simulink library "starslibGeodesy"  (R2022b)
settings: Solver=ode45  StartTime=0.0  StopTime=10.0  RelTol=1e-3  EnableMultiTasking=on
undefined symbols (not defined in the file): SimIn
libraries: $bdroot x6, starslibMathOperations x3, simulink x1, starslibAxisTransformations x1
settings Model: Creator=eheim  LastModifiedBy=macheson
settings SolverCC: AlgebraicLoopSolver=TrustRegion
settings DataIOCC: LimitDataPoints=on  SaveFormat=Array  SignalLoggingSaveFormat=ModelDataLogs  ReturnWorkspaceOutputs=off
settings OptimizationCC: ExpressionDepthLimit=2147483647  LifeSpan=inf
settings DebuggingCC: UnderspecifiedInitializationDetection=Classic  MergeDetectMultiDrivingBlocksExec=none  SolverPrmCheckMsg=warning  FcnCallInpInsideContextMsg=warning  UnconnectedInputMsg=warning  UnconnectedOutputMsg=warning  UnconnectedLineMsg=warning  StateNameClashWarn=warning  SFUnexpectedBacktrackingDiag=warning  SFNoUnconditionalDefaultTransitionDiag=warning  SFExecutionAtInitializationDiag=none  SFMachineParentedDataDiag=warning  ArithmeticOperatorsInVariantConditions=warning
settings HardwareCC: ProdBitPerPointer=32  ProdBitPerSizeT=32  ProdBitPerPtrDiffT=32  ProdLargestAtomicFloat=None  ProdIntDivRoundTo=Undefined  ProdEndianess=Unspecified  ProdWordSize=32  ProdHWDeviceType=32-bit Generic
settings ModelReferenceCC: PropagateSignalLabelsOutOfModel=off
settings SFSimCC: SimUseLocalCustomCode=off  CustomCodeUndefinedFunction=UseInterfaceOnly
settings RTWCC: RTWUseLocalCustomCode=off
settings CodeAppCC: StateflowObjectComments=on
settings GRTTargetCC: TargetLangStandard=C89/C90 (ANSI)  CombineOutputUpdateFcns=off  GRTInterface=on
settings ConfigComp: CovMetricSettings=dw  CovSaveCumulativeToWorkspaceVar=on  CovSaveSingleToWorkspaceVar=on  CovExternalEMLEnable=off  CovSFcnEnable=off

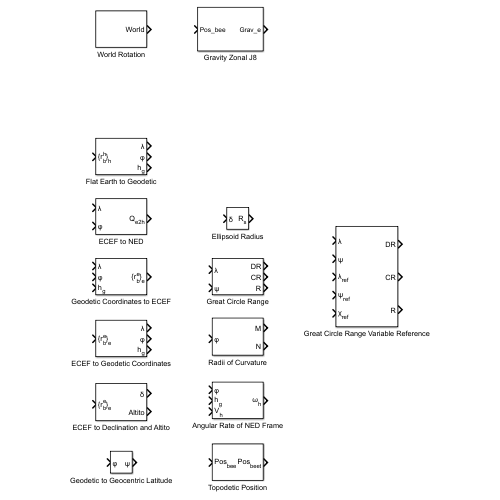
[thumbnail: Simulink's stored preview of the top-level diagram]
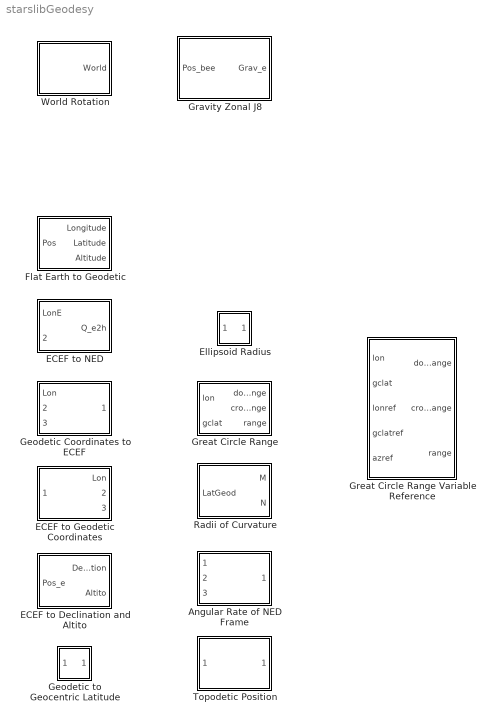
== system starslibGeodesy ==
  Angular Rate of NED Frame : Subsystem  mask(Angular Rate of NED Frame){a=SimIn.Environment.Earth.RadiusEquator, e=SimIn.Environment.Earth.Eccentricity}
      mask prompts: a "Semi-major axis radius"; e "Eccentricity"
      mask help: Computes the angular rate of the local North-East-Down frame.
      mask Display:
      | port_label('input',1,'\phi','texmode','on')
      | port_label('input',2,'h_g','texmode','on')
      | port_label('input',3,'V_h','texmode','on')
      | port_label('output',1,'\omega_{h}','texmode','on')
  ECEF to Declination and Altito : Subsystem  mask(Declination and Altito){a=SimIn.Environment.Earth.RadiusEquator, b=SimIn.Environment.Earth.RadiusPoles}
      mask prompts: a "Semi-major axis radius"; b "Semi-minor axis radius"
      mask help:
      | Calculates angle from equatorial plane to radius vector of vehicle from center of planet, declination and component of radius magnitude above the ellipsoid, altito.
      |
      | Note: Units of input parameters must be same as units of the ECEF position input.
      mask Display:
      | port_label('input',1,'\{r_b^e\}_e','texmode','on')
      | port_label('output',1,'\delta','texmode','on')
      | port_label('output',2,'Altito','texmode','on')
  ECEF to Geodetic Coordinates : Subsystem  mask(ECEF to LLA){a=SimIn.Environment.Earth.RadiusEquator, b=SimIn.Environment.Earth.RadiusPoles, tol=1e-12}
      mask prompts: a "Semi-major axis radius"; b "Semi-minor axis radius"; tol "Minum distance from semi-minor axis"
      mask help:
      | Calculates Longitude, Geodetic Latitude and Geodetic Altitude from Earth Centered Earth Fixed (ECEF) position.
      |
      | Note: Units of input parameters must be same as units of the ECEF position input.
      |
      | Reference:
      | Explanatory Supplement to the Astronomical Almanac
      | Edited by P. Kenneth Seidelmann, 1992
      | University Science Books
      | Sausalito, California
      mask Display:
      | port_label('input',1,'\{r_b^e\}_e','texmode','on')
      | port_label('output',1,'\lambda','texmode','on')
      | port_label('output',2,'\phi','texmode','on')
      | port_label('output',3,'h_g','texmode','on')
  ECEF to NED : Subsystem  mask(ECEF to NED){}
      mask help: Creates quaternion from ECEF axes to local North-East-Down axes by transforming through longitude and geodetic latitude.
      mask Display:
      | port_label('output',1,'Q_{e2h}','texmode','on')
      | port_label('input',1,'\lambda','texmode','on')
      | port_label('input',2,'\phi','texmode','on')
  Ellipsoid Radius : Subsystem  mask(Ellipsoid radius){a=SimIn.Environment.Earth.RadiusEquator, b=SimIn.Environment.Earth.RadiusPoles}
      mask prompts: a "Semi-major axis radius"; b "Semi-minor axis radius"
      mask help: Radius of ellipsoid at geocentric latitude or declination. If geocentric latitude is used the output is the ellipsoid radius at that geocentric latitude. If declination is used the output is then radius of ellipsoid where radius to vehicle pierces the ellipsoid. Units of radius vector are determined by units of semi-major-axis parmeter.
      mask Help:
      | Ref: E. W. PURCELL, E. W. and COWAN, W. B., Relating Geodetic Latitude and Altitude to Geocentric Latitude and Radius Vector, ARS Journal, Jan. 1961, page 934, eqn 5.
      | W. B. COWAN2
      | Aeronutronic Div., Ford Motor Co.
      | Newport Beach, Calif.
      mask Display:
      | port_label('input',1,'\delta','texmode','on')
      | port_label('output',1,'R_s','texmode','on')
  Flat Earth to Geodetic : Subsystem  mask(Flat Earth to Geodetic){lat=SimIn.IC.LatGeod, lon=SimIn.IC.Lon, a=SimIn.Environment.Earth.RadiusEquator, e=SimIn.Environment.Earth.Eccentricity}
      mask prompts: lat "Initial geodetic latitude (radians)"; lon "Initial longitude (radians)"; a "Planet semi-major axis radius"; e "Planet eccentricity"
      mask help: Estimates geodetic latitude, longitude and altitude from change in North-East-Down position. Input position units must match units of planet parmeters.
      mask Display:
      | port_label('input',1,'\{r_b^h\}_h','texmode','on')
      | port_label('output',1,'\lambda','texmode','on')
      | port_label('output',2,'\phi','texmode','on')
      | port_label('output',3,'h_g','texmode','on')
  Geodetic Coordinates to ECEF : Subsystem  mask(LLA to ECEF){a=SimIn.Environment.Earth.RadiusEquator, e=SimIn.Environment.Earth.Eccentricity}
      mask prompts: a "Semi-major axis radius"; e "Eccentricity"
      mask help: Converts geodetic latitude, longitude, and altitude to Cartesian ECEF coordinates.
      mask Display:
      | port_label('output',1,'\{r_b^e\}_e','texmode','on')
      | port_label('input',1,'\lambda','texmode','on')
      | port_label('input',2,'\phi','texmode','on')
      | port_label('input',3,'h_g','texmode','on')
  Geodetic to Geocentric Latitude : Subsystem  mask(Geodetic to Geocentric Latitude){e=SimIn.Environment.Earth.Eccentricity}
      mask prompts: e "Eccentricity"
      mask help: Converts geodetic latitude to geocentric latitude.
      mask Display:
      | port_label('input',1,'\phi','texmode','on')
      | port_label('output',1,'\psi','texmode','on')
  Gravity Zonal J8 : Subsystem  mask(Gravity Zonal J8){a=SimIn.Environment.Earth.RadiusEquator, mu=SimIn.Environment.Earth.Gravity.mu, J=SimIn.Environment.Earth.Gravity.Jcoefs}
      mask prompts: a "Semi-major axis radius"; mu "Gravitational Constant"; J "Zonal Coefficients"
      mask help: Gravity model with up to 8 zonal coefficients.
  Great Circle Range : Subsystem  mask(Great Circle Range){signconv=Positive approaching reference, lonref=SimIn.Environment.Runway.Lon, latref=SimIn.Environment.Runway.LatGeoc, Rref=SimIn.Environment.Runway.Rref, azref=SimIn.Environment.Runway.Heading, a=SimIn.Environment.Earth.RadiusEquator, b=SimIn.Environment.Earth.RadiusPoles}
      mask prompts: signconv "Downrange sign convention"; lonref "Reference Longitude (rad)"; latref "Reference Geocentric Latitude (rad)"; Rref "Refernce Ellipsoid Radius"; azref "Reference Azimuth (rad)"; a "Semi-major-axis radius"; b "Semi-minor-axis radius"
      mask help:
      | Computes downrange and cross range based on relative great circles between the reference location and the vehicle location given longitude and geocentric latitude of each and a reference azimuth.
      |
      | The refernce azimuth can be any arbitrary fixed azimuth.  For example, launch vehicles typically use the launch azimuth with downrange positive departing the reference.  Approach and landing vehicle may use the runway azimuth.
      |
      | Crossrange is defined as the perpendicular distance from the great circle of the reference azimuth to the vehicle.  Cross range is positive in the increasing azimuth direction.
      |
      | Downrange is defined as the distance along the great circle created by the reference azimuth from the reference location to the point at which the crossrange is measured from.  Downrange sign convention can be selected to be either positive when departing or positive when approaching the reference location along the reference azimuth.
      |
      | Units used for Earth radii determine units for downrange and crossrange.
      mask init:
      | switch signconv
      |     case 1
      |         signconv = 1;
      |     case 2
      |         signconv = -1;
      | end
      mask TypeOptions signconv: Positive departing reference | Positive approaching reference
      mask Display:
      | port_label('input',1,'\lambda','texmode','on')
      | port_label('input',2,'\psi','texmode','on')
      | port_label('output',1,'DR','texmode','on')
      | port_label('output',2,'CR','texmode','on')
      | port_label('output',3,'R','texmode','on')
  Great Circle Range Variable Reference : Subsystem  mask(Great Circle Range Variable Reference){signconv=Positive approaching reference, a=SimIn.Environment.Earth.RadiusEquator, b=SimIn.Environment.Earth.RadiusPoles}
      mask prompts: signconv "Downrange sign convention"; a "Semi-major-axis radius"; b "Semi-minor-axis radius"
      mask help:
      | Computes downrange and cross range based on relative great circles between the reference location and the vehicle location given longitude and geocentric latitude of each and a reference azimuth.
      |
      | The refernce azimuth can be any arbitrary azimuth.  For example, launch vehicles typically use the launch azimuth with downrange positive departing the reference.  Approach and landing vehicle may use the runway azimuth or the vehicle ground track with downrange positive approaching the reference location.
      |
      | Crossrange is defined as the perpendicular distance from the great circle of the reference azimuth to the vehicle.  Cross range is positive in the increasing azimuth direction.
      |
      | Downrange is defined as the distance along the great circle created by the reference azimuth from the reference location to the point at which the crossrange is measured from.  Downrange sign convention can be selected to be either positive when departing or positive when approaching the reference location along the reference azimuth.
      |
      | Units used for Earth radii determine units for downrange and crossrange.
      mask init:
      | switch signconv
      |     case 1
      |         signconv = 1;
      |     case 2
      |         signconv = -1;
      | end
      mask TypeOptions signconv: Positive departing reference | Positive approaching reference
      mask Display:
      | port_label('input',1,'\lambda','texmode','on')
      | port_label('input',2,'\psi','texmode','on')
      | port_label('input',3,'\lambda_{ref}','texmode','on')
      | port_label('input',4,'\psi_{ref}','texmode','on')
      | port_label('input',5,'\chi_{ref}','texmode','on')
      | 
      | port_label('output',1,'DR','texmode','on')
      | port_label('output',2,'CR','texmode','on')
      | port_label('output',3,'R','texmode','on')
  Radii of Curvature : Subsystem  mask(Radii of Curvature){a=SimIn.Environment.Earth.RadiusEquator, e=SimIn.Environment.Earth.Eccentricity}
      mask prompts: a "Semi-major axis radius"; e "Eccentricity"
      mask help: Computes the radii of curvature for the ellipsoid
      mask Display:
      | port_label('input',1,'\phi','texmode','on')
      | port_label('output',1,'M','texmode','on')
      | port_label('output',2,'N','texmode','on')
  Topodetic Position : Subsystem  mask(Topodedic Position){Pos_bee=SimIn.EOM.Pos_bee, Q_e2h=SimIn.EOM.Q_e2h}
      mask prompts: Pos_bee "Initial Position (Pos_bee)"; Q_e2h "Initial Transformation (Q_e2h)"
      mask help: NED position relative to initial NED position in initial NED coordinates.
      mask Display:
      | port_label('input' ,1,'Pos_{bee}','texmode','on')
      | port_label('output' ,1,'Pos_{bee}_t','texmode','on')
  World Rotation : Subsystem  mask(World Rotation){omega=SimIn.Environment.Earth.Omega, ERA_IC=SimIn.Environment.Earth.ERA_IC}
      mask prompts: omega "Rotation Rate"; ERA_IC "Initial Rotation Angle"
      mask help:
      | Tracks current world rotation angle and inertial orientation as simulation progresses.
      |
      | Note: The initial rotation angle is for simulation time equal to zero.
      mask Display: port_label('output', 1, 'World');

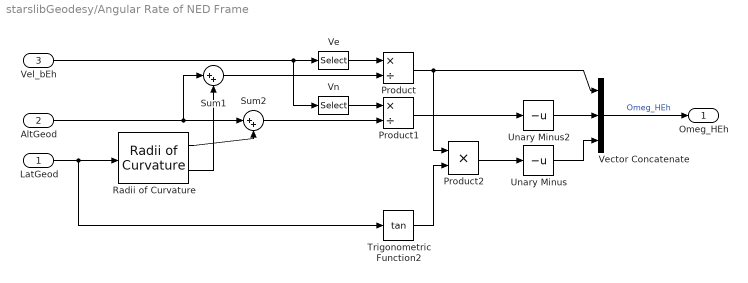
== system starslibGeodesy/Angular Rate of NED Frame ==
  LatGeod : Inport
  AltGeod : Inport  Port=2
  Vel_bEh : Inport  Port=3
  Product : Product  Inputs=*/  RndMeth=Zero
  Product1 : Product  Inputs=*/  RndMeth=Zero
  Product2 : Product  RndMeth=Zero
  Radii of Curvature : $bdroot/Radii of Curvature  a=a  e=e
  Sum1 : Sum  Inputs=|++
  Sum2 : Sum  Inputs=|++
  Trigonometric Function2 : Trigonometry  Operator=tan
  Unary Minus : UnaryMinus
  Unary Minus2 : UnaryMinus
  Ve : Selector  NumberOfDimensions=2  InputPortWidth=3  IndexOptions=Index vector (dialog),Select all  Indices=2,1  OutputSizes=1,1
  Vector Concatenate : Concatenate  NumInputs=3  Mode=Multidimensional array
  Vn : Selector  NumberOfDimensions=2  InputPortWidth=3  IndexOptions=Index vector (dialog),Select all  Indices=1,1  OutputSizes=1,1
  Omeg_HEh : Outport  PortDimensions=[3,1]
  wires:
  Vel_bEh/1 -> Vn/1, Ve/1
  LatGeod/1 -> Radii of Curvature/1, Trigonometric Function2/1
  Trigonometric Function2/1 -> Product2/2
  Vector Concatenate/1 -> Omeg_HEh/1  "Omeg_HEh"
  Product/1 -> Vector Concatenate/1, Product2/1
  Product2/1 -> Unary Minus/1
  Product1/1 -> Unary Minus2/1
  Ve/1 -> Product/1
  Vn/1 -> Product1/1
  Unary Minus2/1 -> Vector Concatenate/2
  Unary Minus/1 -> Vector Concatenate/3
  Sum1/1 -> Product/2
  Sum2/1 -> Product1/2
  Radii of Curvature/2 -> Sum1/2
  Radii of Curvature/1 -> Sum2/2
  AltGeod/1 -> Sum1/1, Sum2/1

== system starslibGeodesy/ECEF to Declination and Altito ==
  Pos_e : Inport
  Ellipsoid Radius : $bdroot/Ellipsoid Radius  a=a  b=b
  Math Function : Math  Operator=hypot  SignedPower=on
  Math Function1 : Math  Operator=hypot  SignedPower=on
  Selector : Selector  InputPortWidth=3  IndexOptions=Index vector (dialog)  Indices=3  OutputSizes=1
  Selector1 : Selector  InputPortWidth=3  IndexOptions=Index vector (dialog)  Indices=2  OutputSizes=1
  Selector2 : Selector  InputPortWidth=3  IndexOptions=Index vector (dialog)  Indices=1  OutputSizes=1
  Sum : Sum  Inputs=|+-
  Trigonometric Function3 : Trigonometry  Operator=atan2
  Declination : Outport
  Altito : Outport  Port=2
  wires:
  Sum/1 -> Altito/1  "Altito"
  Selector1/1 -> Math Function/2
  Selector2/1 -> Math Function/1
  Pos_e/1 -> Selector2/1, Selector/1, Selector1/1
  Math Function/1 -> Trigonometric Function3/2, Math Function1/2
  Selector/1 -> Trigonometric Function3/1, Math Function1/1
  Trigonometric Function3/1 -> Declination/1, Ellipsoid Radius/1  "Declination"
  Math Function1/1 -> Sum/1
  Ellipsoid Radius/1 -> Sum/2

== system starslibGeodesy/ECEF to Geodetic Coordinates ==
  note: Reference:
      | Explanatory Supplement to the Astronomical Almanac
      | Edited by P. Kenneth Seidelmann, 1992
      | University Science Books
      | Sausalito, California
  Pos_bee : Inport
  Distance to Axis : Subsystem
  Geodetic Altitude : Subsystem
  Geodetic Latitude : Subsystem
  Selector2 : Selector  InputPortWidth=3  IndexOptions=Index vector (dialog)  Indices=1  OutputSizes=1
  Selector3 : Selector  InputPortWidth=3  IndexOptions=Index vector (dialog)  Indices=2  OutputSizes=1
  Selector5 : Selector  InputPortWidth=3  IndexOptions=Index vector (dialog)  Indices=3  OutputSizes=1
  Trigonometric Function1 : Trigonometry  Operator=atan2
  t : Subsystem
  Lon : Outport
  LatGeod : Outport  Port=2
  AltGeod : Outport  Port=3
  wires:
  Trigonometric Function1/1 -> Lon/1  "Lon"
  Selector2/1 -> Trigonometric Function1/2  "X"
  Selector3/1 -> Trigonometric Function1/1  "Y"
  Geodetic Altitude/1(AltGeod) -> AltGeod/1  "AltGeod"
  Distance to Axis/1(r) -> Geodetic Altitude/2(r), t/2(r)  "r"
  Geodetic Latitude/1(LatGeod) -> LatGeod/1, Geodetic Altitude/4(LatGeod)  "LatGeod"
  Distance to Axis/2(min) -> Geodetic Latitude/3(min)
  t/1(t) -> Geodetic Altitude/3(t), Geodetic Latitude/2(t)
  Pos_bee/1 -> Selector3/1, Selector2/1, Selector5/1, Distance to Axis/1(Pos)
  Selector5/1 -> t/1(Z), Geodetic Latitude/1(Z), Geodetic Altitude/1(Z)  "Z"

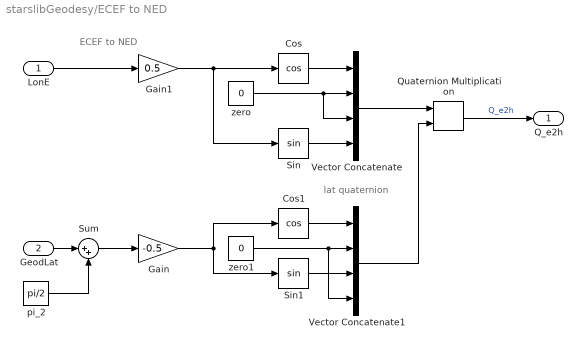
== system starslibGeodesy/ECEF to NED ==
  note: lat quaternion
  note: ECEF to NED
  LonE : Inport
  GeodLat : Inport  Port=2
  Cos : Trigonometry  Operator=cos
  Cos1 : Trigonometry  Operator=cos
  Gain : Gain  Gain=-0.5
  Gain1 : Gain  Gain=0.5
  Quaternion Multiplication : starslibMathOperations/Quaternion Multiplication  n=0
  Sin : Trigonometry
  Sin1 : Trigonometry
  Sum : Sum  Inputs=|++
  Vector Concatenate : Concatenate  NumInputs=4  Mode=Multidimensional array
  Vector Concatenate1 : Concatenate  NumInputs=4  Mode=Multidimensional array
  pi_2 : Constant  Value=pi/2
  zero : Constant  Value=0
  zero1 : Constant  Value=0
  Q_e2h : Outport
  wires:
  GeodLat/1 -> Sum/1
  LonE/1 -> Gain1/1
  Quaternion Multiplication/1 -> Q_e2h/1  "Q_e2h"
  Vector Concatenate1/1 -> Quaternion Multiplication/2
  Vector Concatenate/1 -> Quaternion Multiplication/1
  Gain/1 -> Sin1/1, Cos1/1
  Sin1/1 -> Vector Concatenate1/3
  Cos1/1 -> Vector Concatenate1/1
  Gain1/1 -> Sin/1, Cos/1
  Sin/1 -> Vector Concatenate/4
  zero/1 -> Vector Concatenate/2, Vector Concatenate/3
  Cos/1 -> Vector Concatenate/1
  Sum/1 -> Gain/1
  pi_2/1 -> Sum/2
  zero1/1 -> Vector Concatenate1/2, Vector Concatenate1/4

== system starslibGeodesy/Ellipsoid Radius ==
  Declination : Inport
  Add1 : Sum  Inputs=-+
  Add2 : Sum
  Constant1 : Constant  Value=b
  Constant2 : Constant
  Constant4 : Constant  Value=a
  Divide : Product  Inputs=*/
  Divide1 : Product  Inputs=*/
  Math Function1 : Math  Operator=square  SignedPower=on
  Math Function7 : Math  Operator=square  SignedPower=on
  Product5 : Product  RndMeth=Zero
  Sqrt : Sqrt
  Trigonometric Function : Trigonometry
  Rs : Outport
  wires:
  Trigonometric Function/1 -> Math Function7/1
  Constant2/1 -> Add1/1, Add2/1
  Add1/1 -> Product5/1
  Product5/1 -> Add2/2
  Math Function7/1 -> Product5/2
  Add2/1 -> Sqrt/1
  Sqrt/1 -> Divide/2
  Divide/1 -> Rs/1  "Rs"
  Declination/1 -> Trigonometric Function/1
  Divide1/1 -> Math Function1/1
  Math Function1/1 -> Add1/2
  Constant1/1 -> Divide1/2
  Constant4/1 -> Divide1/1, Divide/1

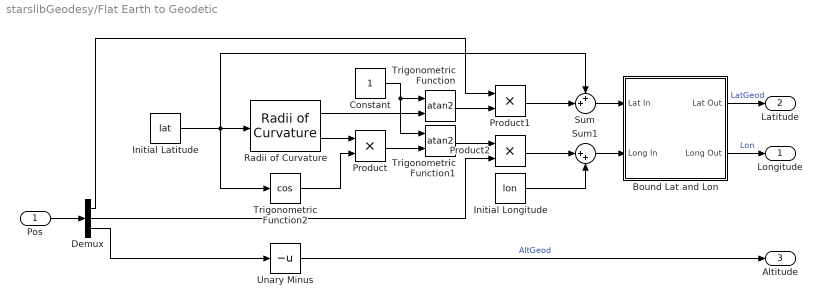
== system starslibGeodesy/Flat Earth to Geodetic ==
  Pos : Inport
  Bound Lat and Lon : Subsystem
  Constant : Constant
  Demux : Demux  Outputs=3
  Initial Latitude : Constant  Value=lat
  Initial Longitude : Constant  Value=lon
  Product : Product  RndMeth=Zero
  Product1 : Product  RndMeth=Zero
  Product2 : Product  RndMeth=Zero
  Radii of Curvature : $bdroot/Radii of Curvature  a=a  e=e
  Sum : Sum  Inputs=++|
  Sum1 : Sum  Inputs=|++
  Trigonometric Function : Trigonometry  Operator=atan2
  Trigonometric Function1 : Trigonometry  Operator=atan2
  Trigonometric Function2 : Trigonometry  Operator=cos
  Unary Minus : UnaryMinus
  Longitude : Outport
  Latitude : Outport  Port=2
  Altitude : Outport  Port=3
  wires:
  Radii of Curvature/2 -> Product/1
  Initial Latitude/1 -> Radii of Curvature/1, Trigonometric Function2/1, Sum/1
  Trigonometric Function2/1 -> Product/2
  Initial Longitude/1 -> Sum1/2
  Trigonometric Function/1 -> Product1/2
  Radii of Curvature/1 -> Trigonometric Function/2
  Constant/1 -> Trigonometric Function/1, Trigonometric Function1/1
  Product/1 -> Trigonometric Function1/2
  Trigonometric Function1/1 -> Product2/1
  Pos/1 -> Demux/1
  Demux/1 -> Product1/1
  Demux/2 -> Product2/2
  Demux/3 -> Unary Minus/1
  Unary Minus/1 -> Altitude/1  "AltGeod"
  Product1/1 -> Sum/2
  Product2/1 -> Sum1/1
  Sum/1 -> Bound Lat and Lon/1(Lat In)
  Sum1/1 -> Bound Lat and Lon/2(Long In)
  Bound Lat and Lon/1(Lat Out) -> Latitude/1  "LatGeod"
  Bound Lat and Lon/2(Long Out) -> Longitude/1  "Lon"

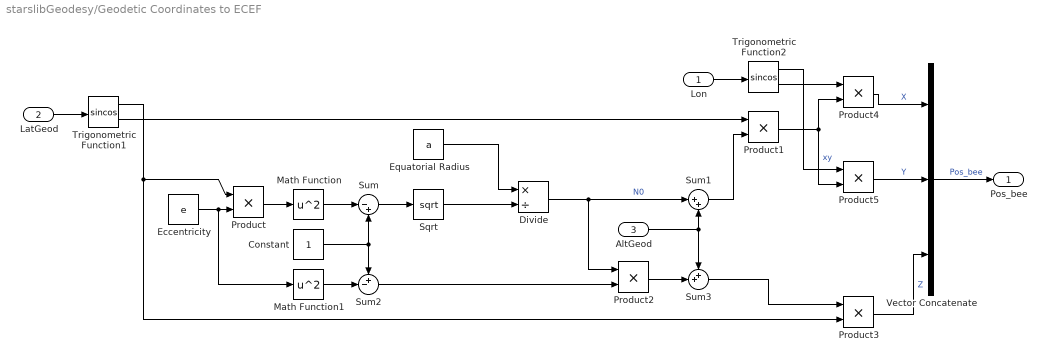
== system starslibGeodesy/Geodetic Coordinates to ECEF ==
  Lon : Inport
  LatGeod : Inport  Port=2
  AltGeod : Inport  Port=3
  Constant : Constant
  Divide : Product  Inputs=*/
  Eccentricity : Constant  Value=e
  Equatorial Radius : Constant  Value=a
  Math Function : Math  Operator=square  SignedPower=on
  Math Function1 : Math  Operator=square  SignedPower=on
  Product{,1..5} (6 alike) : Product  RndMeth=Zero
  Sqrt : Sqrt
  Sum : Sum  Inputs=|-+
  Sum1 : Sum  Inputs=|++
  Sum2 : Sum  Inputs=+-|
  Sum3 : Sum  Inputs=++|
  Trigonometric Function1 : Trigonometry  Operator=sincos
  Trigonometric Function2 : Trigonometry  Operator=sincos
  Vector Concatenate : Concatenate  NumInputs=3  Mode=Multidimensional array
  Pos_bee : Outport
  wires:
  Equatorial Radius/1 -> Divide/1
  Sqrt/1 -> Divide/2
  Eccentricity/1 -> Product/2, Math Function1/1
  Trigonometric Function1/1 -> Product/1, Product3/2
  Product/1 -> Math Function/1
  Constant/1 -> Sum/2, Sum2/1
  Math Function/1 -> Sum/1
  Sum/1 -> Sqrt/1
  Divide/1 -> Sum1/1, Product2/1  "N0"
  AltGeod/1 -> Sum1/2, Sum3/1
  Sum1/1 -> Product1/2
  Product1/1 -> Product4/2, Product5/2  "xy"
  Math Function1/1 -> Sum2/2
  Sum2/1 -> Product2/2
  LatGeod/1 -> Trigonometric Function1/1
  Trigonometric Function1/2 -> Product1/1
  Trigonometric Function2/1 -> Product5/1
  Trigonometric Function2/2 -> Product4/1
  Lon/1 -> Trigonometric Function2/1
  Product5/1 -> Vector Concatenate/2  "Y"
  Product4/1 -> Vector Concatenate/1  "X"
  Product3/1 -> Vector Concatenate/3  "Z"
  Vector Concatenate/1 -> Pos_bee/1  "Pos_bee"
  Product2/1 -> Sum3/2
  Sum3/1 -> Product3/1

== system starslibGeodesy/Geodetic to Geocentric Latitude ==
  Geodetic Latitude : Inport
  Constant : Constant
  Constant1 : Constant  Value=e
  Math Function : Math  Operator=square  SignedPower=on
  Product : Product
  Sum : Sum  Inputs=|+-
  Trigonometric Function : Trigonometry  Operator=tan
  Trigonometric Function1 : Trigonometry  Operator=atan
  Geocentric Latitude : Outport
  wires:
  Product/1 -> Trigonometric Function1/1
  Trigonometric Function/1 -> Product/1
  Trigonometric Function1/1 -> Geocentric Latitude/1
  Geodetic Latitude/1 -> Trigonometric Function/1
  Constant/1 -> Sum/1
  Sum/1 -> Product/2
  Constant1/1 -> Math Function/1
  Math Function/1 -> Sum/2

== system starslibGeodesy/Gravity Zonal J8 ==
  Pos_bee : Inport
  Constant : Constant  Value=a
  Constant1 : Constant  Value=mu
  Constant2 : Constant  Value=J
  Gravity Zonal J8 : MATLAB Function  TreatAsAtomicUnit=on
  Grav_e : Outport
  wires:
  Pos_bee/1 -> Gravity Zonal J8/1(pecef)
  Constant2/1 -> Gravity Zonal J8/4(J)
  Constant1/1 -> Gravity Zonal J8/3(mu)
  Constant/1 -> Gravity Zonal J8/2(a)
  Gravity Zonal J8/1(Grav_e) -> Grav_e/1  "Grav_e"

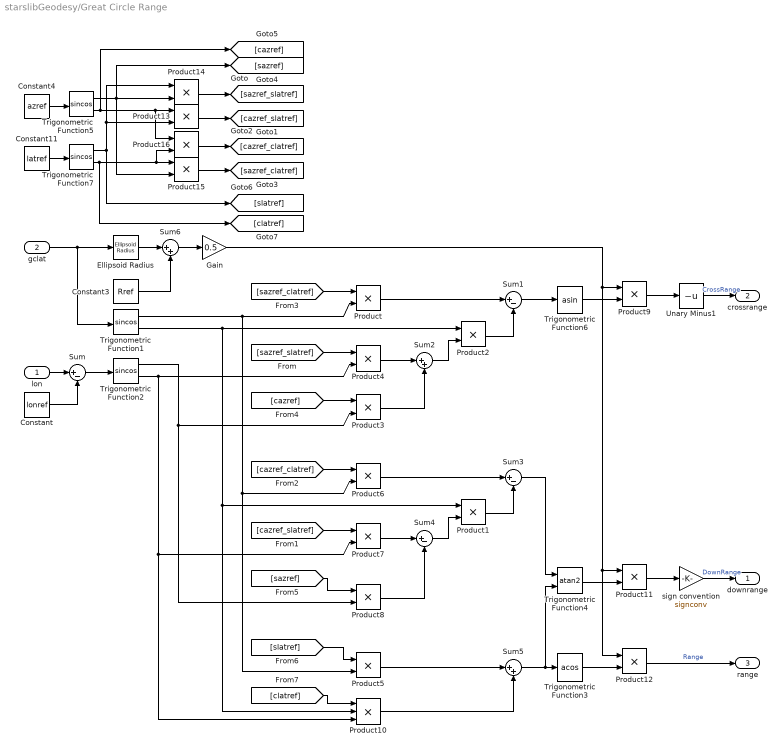
== system starslibGeodesy/Great Circle Range ==
  lon : Inport
  gclat : Inport  Port=2
  Constant : Constant  Value=lonref
  Constant11 : Constant  Value=latref
  Constant3 : Constant  Value=Rref
  Constant4 : Constant  Value=azref
  Ellipsoid Radius : $bdroot/Ellipsoid Radius  a=a  b=b
  Gain : Gain  Gain=0.5
  Product{,1..9,11..16} (16 alike) : Product  RndMeth=Zero
  Product10 : Product  Inputs=3  RndMeth=Zero
  Sum{,1,3..4} (4 alike) : Sum  Inputs=|+-
  Sum2 : Sum  Inputs=|++
  Sum5 : Sum  Inputs=|++
  Sum6 : Sum  Inputs=|++
  Trigonometric Function{1..2,5,7} (4 alike) : Trigonometry  Operator=sincos
  Trigonometric Function3 : Trigonometry  Operator=acos
  Trigonometric Function4 : Trigonometry  Operator=atan2
  Trigonometric Function6 : Trigonometry  Operator=asin
  Unary Minus1 : UnaryMinus
  sign convention : Gain  Gain=signconv
  downrange : Outport
  crossrange : Outport  Port=2
  range : Outport  Port=3
  wires:
  Constant/1 -> Sum/2
  lon/1 -> Sum/1
  Sum/1 -> Trigonometric Function2/1
  [sazref_clatref] -> Product/1
  [sazref_slatref] -> Product4/1
  gclat/1 -> Trigonometric Function1/1, Ellipsoid Radius/1
  Product/1 -> Sum1/1
  Product4/1 -> Sum2/1
  Trigonometric Function2/2 -> Product4/2, Product10/3, Product7/2
  [cazref] -> Product3/1
  Trigonometric Function2/1 -> Product3/2, Product8/2
  Trigonometric Function1/1 -> Product/2, Product6/2, Product5/2
  [cazref_clatref] -> Product6/1
  [cazref_slatref] -> Product7/1
  Product6/1 -> Sum3/1
  Product7/1 -> Sum4/1
  [sazref] -> Product8/1
  Product8/1 -> Sum4/2
  [slatref] -> Product5/1
  [clatref] -> Product10/1
  Product5/1 -> Sum5/1
  Product10/1 -> Sum5/2
  Sum2/1 -> Product2/2
  Product2/1 -> Sum1/2
  Trigonometric Function1/2 -> Product2/1, Product1/1, Product10/2
  Sum4/1 -> Product1/2
  Product1/1 -> Sum3/2
  Product3/1 -> Sum2/2
  Ellipsoid Radius/1 -> Sum6/1
  Constant3/1 -> Sum6/2
  Sum6/1 -> Gain/1
  Sum1/1 -> Trigonometric Function6/1
  Sum3/1 -> Trigonometric Function4/1
  Sum5/1 -> Trigonometric Function4/2, Trigonometric Function3/1
  Trigonometric Function4/1 -> Product11/2
  Trigonometric Function6/1 -> Product9/2
  Gain/1 -> Product9/1, Product11/1, Product12/1
  Product9/1 -> Unary Minus1/1
  Product11/1 -> sign convention/1
  Unary Minus1/1 -> crossrange/1  "CrossRange"
  sign convention/1 -> downrange/1  "DownRange"
  Trigonometric Function3/1 -> Product12/2
  Product12/1 -> range/1  "Range"
  Constant4/1 -> Trigonometric Function5/1
  Constant11/1 -> Trigonometric Function7/1
  Trigonometric Function5/2 -> [cazref], Product16/1, Product13/1
  Trigonometric Function5/1 -> [sazref], Product15/2, Product14/2
  Trigonometric Function7/1 -> Product13/2, Product14/1, [slatref]
  Trigonometric Function7/2 -> [clatref], Product16/2, Product15/1
  Product14/1 -> [sazref_slatref]
  Product13/1 -> [cazref_slatref]
  Product16/1 -> [cazref_clatref]
  Product15/1 -> [sazref_clatref]

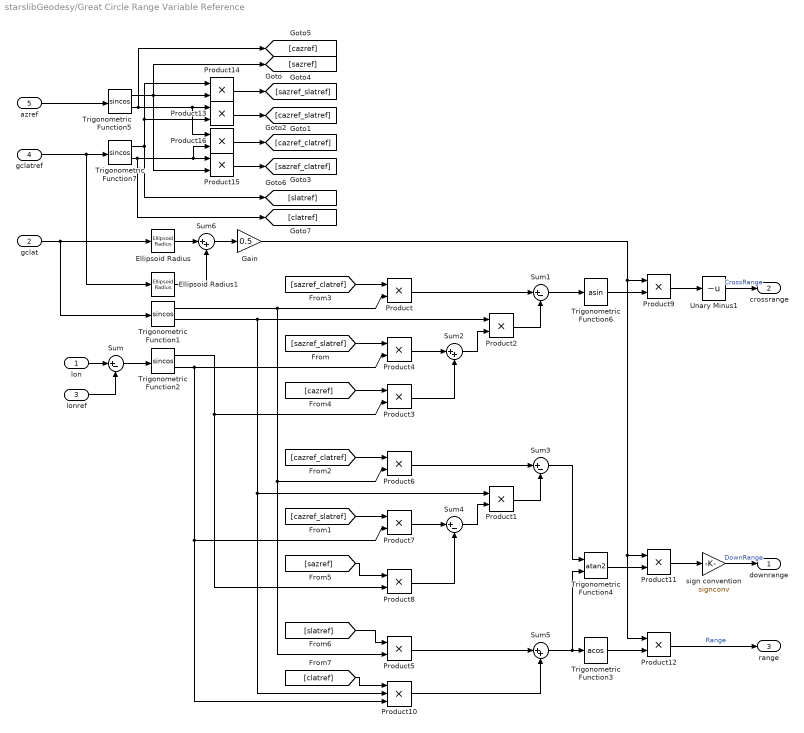
== system starslibGeodesy/Great Circle Range Variable Reference ==
  lon : Inport
  gclat : Inport  Port=2
  lonref : Inport  Port=3
  gclatref : Inport  Port=4
  azref : Inport  Port=5
  Ellipsoid Radius : $bdroot/Ellipsoid Radius  a=a  b=b
  Ellipsoid Radius1 : $bdroot/Ellipsoid Radius  a=a  b=b
  Gain : Gain  Gain=0.5
  Product{,1..9,11..16} (16 alike) : Product  RndMeth=Zero
  Product10 : Product  Inputs=3  RndMeth=Zero
  Sum{,1,3..4} (4 alike) : Sum  Inputs=|+-
  Sum2 : Sum  Inputs=|++
  Sum5 : Sum  Inputs=|++
  Sum6 : Sum  Inputs=|++
  Trigonometric Function{1..2,5,7} (4 alike) : Trigonometry  Operator=sincos
  Trigonometric Function3 : Trigonometry  Operator=acos
  Trigonometric Function4 : Trigonometry  Operator=atan2
  Trigonometric Function6 : Trigonometry  Operator=asin
  Unary Minus1 : UnaryMinus
  sign convention : Gain  Gain=signconv
  downrange : Outport
  crossrange : Outport  Port=2
  range : Outport  Port=3
  wires:
  Product15/1 -> [sazref_clatref]
  Product16/1 -> [cazref_clatref]
  Product13/1 -> [cazref_slatref]
  Product14/1 -> [sazref_slatref]
  Trigonometric Function7/2 -> Product15/1, Product16/2, [clatref]
  Trigonometric Function7/1 -> [slatref], Product14/1, Product13/2
  Trigonometric Function5/1 -> Product14/2, Product15/2, [sazref]
  Trigonometric Function5/2 -> Product13/1, Product16/1, [cazref]
  gclatref/1 -> Ellipsoid Radius1/1, Trigonometric Function7/1
  azref/1 -> Trigonometric Function5/1
  Product12/1 -> range/1  "Range"
  Trigonometric Function3/1 -> Product12/2
  sign convention/1 -> downrange/1  "DownRange"
  Unary Minus1/1 -> crossrange/1  "CrossRange"
  Product11/1 -> sign convention/1
  Product9/1 -> Unary Minus1/1
  Gain/1 -> Product12/1, Product11/1, Product9/1
  Trigonometric Function6/1 -> Product9/2
  Trigonometric Function4/1 -> Product11/2
  Sum5/1 -> Trigonometric Function3/1, Trigonometric Function4/2
  Sum3/1 -> Trigonometric Function4/1
  Sum1/1 -> Trigonometric Function6/1
  Sum6/1 -> Gain/1
  Ellipsoid Radius1/1 -> Sum6/2
  Ellipsoid Radius/1 -> Sum6/1
  Product3/1 -> Sum2/2
  Product1/1 -> Sum3/2
  Sum4/1 -> Product1/2
  Trigonometric Function1/2 -> Product10/2, Product1/1, Product2/1
  Product2/1 -> Sum1/2
  Sum2/1 -> Product2/2
  Product10/1 -> Sum5/2
  Product5/1 -> Sum5/1
  [clatref] -> Product10/1
  [slatref] -> Product5/1
  Product8/1 -> Sum4/2
  [sazref] -> Product8/1
  Product7/1 -> Sum4/1
  Product6/1 -> Sum3/1
  [cazref_slatref] -> Product7/1
  [cazref_clatref] -> Product6/1
  Trigonometric Function1/1 -> Product5/2, Product6/2, Product/2
  Trigonometric Function2/1 -> Product8/2, Product3/2
  [cazref] -> Product3/1
  Trigonometric Function2/2 -> Product7/2, Product10/3, Product4/2
  Product4/1 -> Sum2/1
  Product/1 -> Sum1/1
  gclat/1 -> Ellipsoid Radius/1, Trigonometric Function1/1
  [sazref_slatref] -> Product4/1
  [sazref_clatref] -> Product/1
  Sum/1 -> Trigonometric Function2/1
  lon/1 -> Sum/1
  lonref/1 -> Sum/2

== system starslibGeodesy/Radii of Curvature ==
  note: Ref: Stevens, B. L. and Lewis, F. L., Aircraft Control and Simulation, 2nd Ed., 2003
      | Eqn. 1.4-3 and 1.4-5
  LatGeod : Inport
  Constant1 : Constant  Value=e
  Constant2 : Constant
  Constant3 : Constant  Value=a
  Math Function1 : Math  Operator=square  SignedPower=on
  Math Function2 : Math  Operator=square  SignedPower=on
  Product3 : Product  Inputs=*/  RndMeth=Zero
  Product4 : Product  RndMeth=Zero
  Product5 : Product  Inputs=**/  RndMeth=Zero
  Sqrt2 : Sqrt
  Sum1 : Sum  Inputs=|+-
  Sum3 : Sum  Inputs=|+-
  Trigonometric Function1 : Trigonometry
  M : Outport
  N : Outport  Port=2
  wires:
  LatGeod/1 -> Trigonometric Function1/1
  Constant1/1 -> Math Function1/1
  Product5/1 -> M/1
  Constant3/1 -> Product3/1
  Sum1/1 -> Product5/1
  Product3/1 -> N/1, Product5/2
  Sqrt2/1 -> Product3/2
  Sum3/1 -> Product5/3, Sqrt2/1
  Product4/1 -> Sum3/2
  Math Function2/1 -> Product4/2
  Trigonometric Function1/1 -> Math Function2/1
  Math Function1/1 -> Product4/1, Sum1/2
  Constant2/1 -> Sum3/1, Sum1/1

== system starslibGeodesy/Topodetic Position ==
  note: Topodedic Position, NED position relative to initial
      | NED position in initial NED coordinates.
  Pos_bee : Inport
  Initial Position : Constant  Value=Pos_bee  VectorParams1D=off
  Initial Transformation : Constant  Value=Q_e2h  VectorParams1D=off
  Quaternion Vector Transformation1 : starslibAxisTransformations/Quaternion Vector Transformation  n=0
  Subtract : Sum  Inputs=+-
  Pos_topo : Outport
  wires:
  Subtract/1 -> Quaternion Vector Transformation1/2
  Initial Transformation/1 -> Quaternion Vector Transformation1/1
  Initial Position/1 -> Subtract/2
  Pos_bee/1 -> Subtract/1
  Quaternion Vector Transformation1/1 -> Pos_topo/1  "Pos_beh_topo"

== system starslibGeodesy/World Rotation ==
  Bus Creator1 : BusCreator  Inputs=3
  Clock : Clock
  ERA_IC_rad : Constant  Value=ERA_IC
  OmegaEarth_rps : Constant  Value=omega
  Product : Product  RndMeth=Zero
  Sum : Sum  Inputs=|++
  Z rotation : Subsystem
  vector : Gain  Gain=[0 0 1]'
  World : Outport
  wires:
  Bus Creator1/1 -> World/1
  ERA_IC_rad/1 -> Sum/2
  Product/1 -> Sum/1
  Clock/1 -> Product/2
  OmegaEarth_rps/1 -> Product/1, vector/1  "rate"
  Sum/1 -> Z rotation/1(angle), Bus Creator1/2  "ERA"
  Z rotation/1(Q) -> Bus Creator1/3  "Q_i2e"
  vector/1 -> Bus Creator1/1  "Omeg_EIi"

== system starslibGeodesy/ECEF to Geodetic Coordinates/Distance to Axis ==
  Pos : Inport
  Compare To Zero : simulink/Logic and Bit Operations/Compare To Zero  relop=>  OutDataTypeStr=boolean  ZeroCross=off
  Math Function : Math  Operator=hypot  SignedPower=on
  Minum Distance From Axis : Constant  Value=tol
  Selector2 : Selector  InputPortWidth=3  IndexOptions=Index vector (dialog)  Indices=1  OutputSizes=1
  Selector3 : Selector  InputPortWidth=3  IndexOptions=Index vector (dialog)  Indices=2  OutputSizes=1
  Subtract : Sum  Inputs=+-
  Switch : Switch  Criteria=u2 ~= 0  Threshold=0.5  ZeroCross=off  SaturateOnIntegerOverflow=off  InputSameDT=off
  r : Outport
  min : Outport  Port=2
  wires:
  Selector2/1 -> Math Function/2
  Selector3/1 -> Math Function/1
  Pos/1 -> Selector2/1, Selector3/1
  Switch/1 -> r/1  "r"
  Minum Distance From Axis/1 -> Switch/3, Subtract/2
  Subtract/1 -> Compare To Zero/1
  Compare To Zero/1 -> min/1, Switch/2
  Math Function/1 -> Subtract/1, Switch/1  "r"

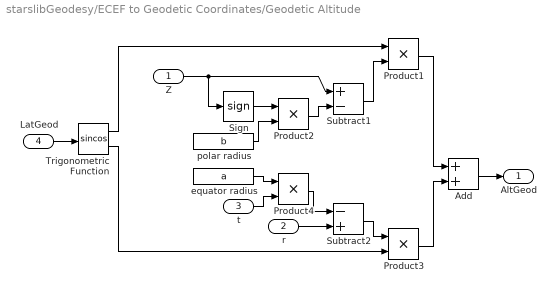
== system starslibGeodesy/ECEF to Geodetic Coordinates/Geodetic Altitude ==
  Z : Inport
  r : Inport  Port=2
  t : Inport  Port=3
  LatGeod : Inport  Port=4
  Add : Sum
  Product{1..4} (4 alike) : Product  RndMeth=Zero
  Sign : Signum
  Subtract1 : Sum  Inputs=+-
  Subtract2 : Sum  Inputs=-+
  Trigonometric Function : Trigonometry  Operator=sincos
  equator radius : Constant  Value=a
  polar radius : Constant  Value=b
  AltGeod : Outport
  wires:
  LatGeod/1 -> Trigonometric Function/1
  Add/1 -> AltGeod/1
  r/1 -> Subtract2/2
  t/1 -> Product4/2
  equator radius/1 -> Product4/1
  polar radius/1 -> Product2/2
  Z/1 -> Sign/1, Subtract1/1
  Product3/1 -> Add/2
  Product1/1 -> Add/1
  Product4/1 -> Subtract2/1
  Subtract2/1 -> Product3/1
  Trigonometric Function/2 -> Product3/2
  Product2/1 -> Subtract1/2
  Sign/1 -> Product2/1
  Subtract1/1 -> Product1/2
  Trigonometric Function/1 -> Product1/1

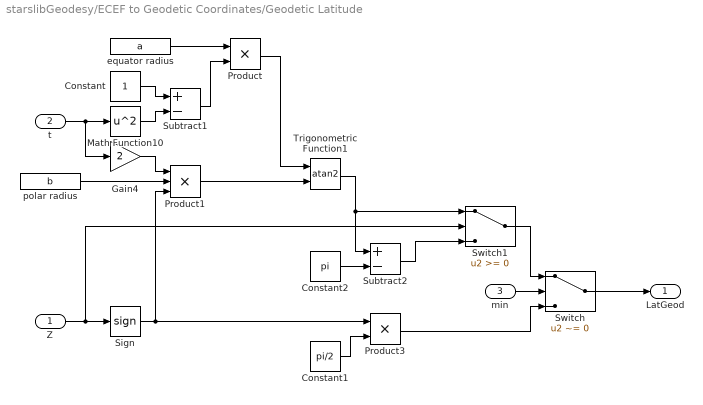
== system starslibGeodesy/ECEF to Geodetic Coordinates/Geodetic Latitude ==
  Z : Inport
  t : Inport  Port=2
  min : Inport  Port=3
  Constant : Constant
  Constant1 : Constant  Value=pi/2
  Constant2 : Constant  Value=pi
  Gain4 : Gain  Gain=2
  Math Function10 : Math  Operator=square  SignedPower=on
  Product : Product  RndMeth=Zero
  Product1 : Product  Inputs=3  RndMeth=Zero
  Product3 : Product  RndMeth=Zero
  Sign : Signum
  Subtract1 : Sum  Inputs=+-
  Subtract2 : Sum  Inputs=+-
  Switch : Switch  Criteria=u2 ~= 0  Threshold=0.5  ZeroCross=off  SaturateOnIntegerOverflow=off  InputSameDT=off
  Switch1 : Switch  ZeroCross=off  SaturateOnIntegerOverflow=off  InputSameDT=off
  Trigonometric Function1 : Trigonometry  Operator=atan2
  equator radius : Constant  Value=a
  polar radius : Constant  Value=b
  LatGeod : Outport
  wires:
  Subtract2/1 -> Switch1/3
  Trigonometric Function1/1 -> Subtract2/1, Switch1/1
  Switch1/1 -> Switch/1
  Constant2/1 -> Subtract2/2
  Switch/1 -> LatGeod/1
  Product/1 -> Trigonometric Function1/1
  Product1/1 -> Trigonometric Function1/2
  min/1 -> Switch/2
  polar radius/1 -> Product1/2
  equator radius/1 -> Product/1
  Constant1/1 -> Product3/2
  Product3/1 -> Switch/3
  Sign/1 -> Product3/1, Product1/3
  Z/1 -> Switch1/2, Sign/1
  Gain4/1 -> Product1/1
  Subtract1/1 -> Product/2
  t/1 -> Math Function10/1, Gain4/1
  Math Function10/1 -> Subtract1/2
  Constant/1 -> Subtract1/1

== system starslibGeodesy/ECEF to Geodetic Coordinates/t ==
  Z : Inport
  r : Inport  Port=2
  E and F : Subsystem
  "t " : Subsystem
  v : Subsystem
  t : Outport
  wires:
  "t "/1(t) -> t/1
  r/1 -> E and F/2(r)
  Z/1 -> E and F/1(Z)
  v/1(v) -> "t "/3(v)
  E and F/2(F) -> "t "/2(F), v/2(F)
  E and F/1(E) -> "t "/1(E), v/1(E)

== system starslibGeodesy/Flat Earth to Geodetic/Bound Lat and Lon ==
  note: Wrap latitude and longitude to +/-90 and +/-180.
  Lat In : Inport
  Long In : Inport  Port=2
  Abs : Abs  SaturateOnIntegerOverflow=off
  Constant : Constant  Value=pi
  Product : Product  RndMeth=Zero
  Sign : Signum
  Sum : Sum  Inputs=|+-
  Sum1 : Sum  Inputs=++|
  Switch1 : Switch  Criteria=u2 > Threshold  Threshold=pi/2  SaturateOnIntegerOverflow=off  InputSameDT=off
  Switch2 : Switch  Criteria=u2 > Threshold  Threshold=pi/2  SaturateOnIntegerOverflow=off  InputSameDT=off
  Wrap : starslibMathOperations/Wrap  R=2*pi  M=-pi
  Wrap1 : starslibMathOperations/Wrap  R=2*pi  M=-pi
  Lat Out : Outport
  Long Out : Outport  Port=2
  wires:
  Wrap1/1 -> Long Out/1
  Abs/1 -> Switch2/2, Switch1/2, Sum/2
  Wrap/1 -> Switch1/3, Abs/1, Sign/1
  Long In/1 -> Switch2/3, Sum1/2
  Switch2/1 -> Wrap1/1
  Constant/1 -> Sum/1, Sum1/1
  Sum/1 -> Product/2
  Sign/1 -> Product/1
  Product/1 -> Switch1/1
  Sum1/1 -> Switch2/1
  Switch1/1 -> Lat Out/1
  Lat In/1 -> Wrap/1

== system starslibGeodesy/World Rotation/Z rotation ==
  angle : Inport
  Constant : Constant  Value=0
  Gain : Gain  Gain=0.5
  Trigonometric Function : Trigonometry
  Trigonometric Function1 : Trigonometry  Operator=cos
  Vector Concatenate : Concatenate  NumInputs=4  Mode=Multidimensional array
  Q : Outport  PortDimensions=[4,1]
  wires:
  Gain/1 -> Trigonometric Function/1, Trigonometric Function1/1
  Trigonometric Function1/1 -> Vector Concatenate/1
  Constant/1 -> Vector Concatenate/2, Vector Concatenate/3
  Trigonometric Function/1 -> Vector Concatenate/4
  angle/1 -> Gain/1
  Vector Concatenate/1 -> Q/1

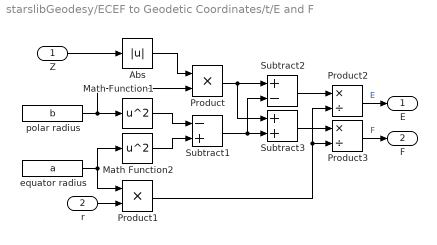
== system starslibGeodesy/ECEF to Geodetic Coordinates/t/E and F ==
  Z : Inport
  r : Inport  Port=2
  Abs : Abs  SaturateOnIntegerOverflow=off
  Math Function1 : Math  Operator=square  SignedPower=on
  Math Function2 : Math  Operator=square  SignedPower=on
  Product : Product  RndMeth=Zero
  Product1 : Product  RndMeth=Zero
  Product2 : Product  Inputs=*/  RndMeth=Zero
  Product3 : Product  Inputs=*/  RndMeth=Zero
  Subtract1 : Sum  Inputs=-+
  Subtract2 : Sum  Inputs=+-
  Subtract3 : Sum
  equator radius : Constant  Value=a
  polar radius : Constant  Value=b
  E : Outport
  F : Outport  Port=2
  wires:
  r/1 -> Product1/2
  Product3/1 -> F/1  "F"
  Product2/1 -> E/1  "E"
  Z/1 -> Abs/1
  Product1/1 -> Product3/2, Product2/2
  Subtract3/1 -> Product3/1
  Subtract2/1 -> Product2/1
  Subtract1/1 -> Subtract2/2, Subtract3/2
  Product/1 -> Subtract3/1, Subtract2/1
  equator radius/1 -> Product1/1, Math Function2/1
  Math Function2/1 -> Subtract1/2
  Math Function1/1 -> Subtract1/1
  polar radius/1 -> Math Function1/1, Product/2
  Abs/1 -> Product/1

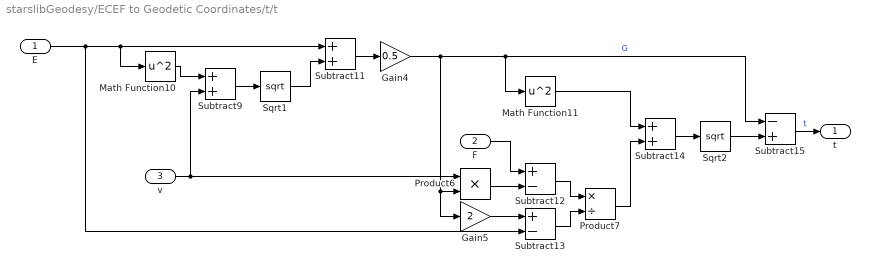
== system starslibGeodesy/ECEF to Geodetic Coordinates/t/t  ==
  E : Inport
  F : Inport  Port=2
  v : Inport  Port=3
  Gain4 : Gain  Gain=0.5
  Gain5 : Gain  Gain=2
  Math Function10 : Math  Operator=square  SignedPower=on
  Math Function11 : Math  Operator=square  SignedPower=on
  Product6 : Product  RndMeth=Zero
  Product7 : Product  Inputs=*/  RndMeth=Zero
  Sqrt1 : Sqrt
  Sqrt2 : Sqrt
  Subtract11 : Sum
  Subtract12 : Sum  Inputs=+-
  Subtract13 : Sum  Inputs=+-
  Subtract14 : Sum
  Subtract15 : Sum  Inputs=-+
  Subtract9 : Sum
  t : Outport
  wires:
  Subtract15/1 -> t/1  "t"
  F/1 -> Subtract12/1
  E/1 -> Subtract13/2, Math Function10/1, Subtract11/1
  Sqrt2/1 -> Subtract15/2
  Subtract14/1 -> Sqrt2/1
  Gain5/1 -> Subtract13/1
  Product6/1 -> Subtract12/2
  Product7/1 -> Subtract14/2
  Math Function11/1 -> Subtract14/1
  Subtract13/1 -> Product7/2
  Subtract12/1 -> Product7/1
  Gain4/1 -> Gain5/1, Product6/2, Math Function11/1, Subtract15/1  "G"
  Subtract11/1 -> Gain4/1
  Sqrt1/1 -> Subtract11/2
  Subtract9/1 -> Sqrt1/1
  Math Function10/1 -> Subtract9/1
  v/1 -> Subtract9/2, Product6/1

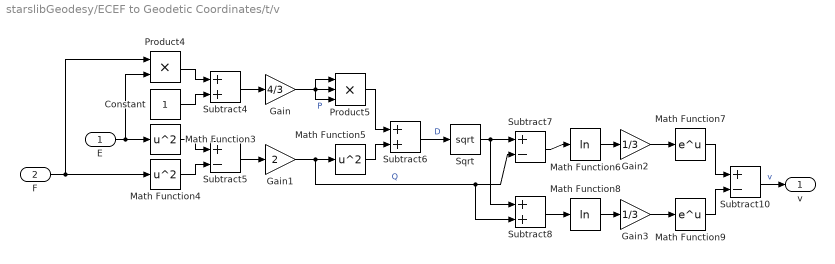
== system starslibGeodesy/ECEF to Geodetic Coordinates/t/v ==
  E : Inport
  F : Inport  Port=2
  Constant : Constant
  Gain : Gain  Gain=4/3
  Gain1 : Gain  Gain=2
  Gain2 : Gain  Gain=1/3
  Gain3 : Gain  Gain=1/3
  Math Function3 : Math  Operator=square  SignedPower=on
  Math Function4 : Math  Operator=square  SignedPower=on
  Math Function5 : Math  Operator=square  SignedPower=on
  Math Function6 : Math  Operator=log  SignedPower=on
  Math Function7 : Math  SignedPower=on
  Math Function8 : Math  Operator=log  SignedPower=on
  Math Function9 : Math  SignedPower=on
  Product4 : Product  RndMeth=Zero
  Product5 : Product  Inputs=3  RndMeth=Zero
  Sqrt : Sqrt
  Subtract10 : Sum  Inputs=+-
  Subtract4 : Sum
  Subtract5 : Sum  Inputs=+-
  Subtract6 : Sum
  Subtract7 : Sum  Inputs=+-
  Subtract8 : Sum
  v : Outport
  wires:
  Subtract10/1 -> v/1  "v"
  F/1 -> Math Function4/1, Product4/1
  E/1 -> Product4/2, Math Function3/1
  Math Function9/1 -> Subtract10/2
  Math Function7/1 -> Subtract10/1
  Gain3/1 -> Math Function9/1
  Gain2/1 -> Math Function7/1
  Subtract8/1 -> Math Function8/1
  Math Function8/1 -> Gain3/1
  Math Function6/1 -> Gain2/1
  Subtract7/1 -> Math Function6/1
  Sqrt/1 -> Subtract8/1, Subtract7/1
  Subtract6/1 -> Sqrt/1  "D"
  Math Function5/1 -> Subtract6/2
  Product5/1 -> Subtract6/1
  Gain1/1 -> Subtract8/2, Subtract7/2, Math Function5/1  "Q"
  Gain/1 -> Product5/3, Product5/1, Product5/2  "P"
  Subtract5/1 -> Gain1/1
  Math Function4/1 -> Subtract5/2
  Math Function3/1 -> Subtract5/1
  Subtract4/1 -> Gain/1
  Constant/1 -> Subtract4/2
  Product4/1 -> Subtract4/1

== matlab function starslibGeodesy/Gravity Zonal J8/Gravity Zonal J8 ==
  data: pecef input; Grav_e output size=[3 1]; a input; mu input; J input
function Grav_e = zonalGrav(pecef,a,mu,J)
%#codegen

% Place-holder for calling Matlab routine in library.

Grav_e = J8Grav(pecef,a,mu,J);
